simulink model "Motor_Diesel_paC"  (R2017a)
settings: Solver=FixedStepAuto  StartTime=0.0  StopTime=1000  FixedStep=0.01  RelTol=1e-3  EnableMultiTasking=on
undefined symbols (not defined in the file): H_act_d, K1
settings Model: Creator=dmartinez  LastModifiedBy=Administrador
settings OptimizationCC: DefaultParameterBehavior=Inlined  PassReuseOutputArgsAs=Individual arguments
settings DebuggingCC: ParameterTunabilityLossMsg=error  SFUnexpectedBacktrackingDiag=warning  SFNoUnconditionalDefaultTransitionDiag=warning  SFExecutionAtInitializationDiag=none
settings SFSimCC: MATLABDynamicMemAlloc=off
settings RTWCC: SystemTargetFile=ert.tlc  TemplateMakefile=ert_default_tmf  Description=Embedded Coder  GenerateReport=on  Toolchain=GNU GCC Raspberry Pi  IncludeHyperlinkInReport=on  LaunchReport=on  GenerateTraceInfo=on  GenerateTraceReport=on  GenerateTraceReportSl=on  GenerateTraceReportSf=on  GenerateTraceReportEml=on
settings CodeAppCC: ForceParamTrailComments=on  IgnoreCustomStorageClasses=off  OperatorAnnotations=on  SimulinkDataObjDesc=on  SFDataObjDesc=on  MATLABFcnDesc=on  InsertBlockDesc=on  MATLABSourceComments=on
settings ERTTargetCC: GenerateSampleERTMain=on  InlinedParameterPlacement=NonHierarchical  ERTCustomFileTemplate=example_file_process.tlc
settings ConfigComp: CovMetricSettings=dw  CovHtmlReporting=on  CovSaveCumulativeToWorkspaceVar=on  CovSaveSingleToWorkspaceVar=on  CovExternalEMLEnable=off

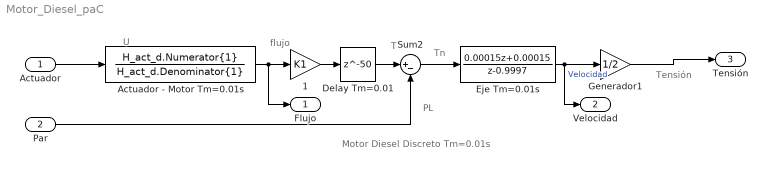
== system Motor_Diesel_paC ==
  note: flujo
  note: T
  note: U
  note: PL
  note: Tn
  note: Motor Diesel Discreto Tm=0.01s
  note: Tensión
  Actuador : Inport  SampleTime=0.01
  Par : Inport  Port=2  SampleTime=0.01
  " 1" : Gain  Gain=K1
  " Generador1" : Gain  Gain=1/2
  Actuador - Motor Tm=0.01s : DiscreteTransferFcn  Numerator=H_act_d.Numerator{1}  Denominator=H_act_d.Denominator{1}  SampleTime=0.01
  Delay Tm=0.01 : Delay  DelayLength=50  SampleTime=0.01
  Eje Tm=0.01s : DiscreteTransferFcn  Numerator=[0.00015 0.00015]  Denominator=[1 -0.9997]  SampleTime=0.01
  Sum2 : Sum  Inputs=|+-
  Flujo : Outport  SampleTime=0.01
  Velocidad : Outport  Port=2  SampleTime=0.01
  Tensión : Outport  Port=3  SampleTime=0.01
  wires:
  Sum2/1 -> Eje Tm=0.01s/1
  Eje Tm=0.01s/1 -> Velocidad/1, " Generador1"/1  "Velocidad"
  Actuador/1 -> Actuador - Motor Tm=0.01s/1
  " Generador1"/1 -> Tensión/1
  Par/1 -> Sum2/2
  Actuador - Motor Tm=0.01s/1 -> " 1"/1, Flujo/1
  " 1"/1 -> Delay Tm=0.01/1
  Delay Tm=0.01/1 -> Sum2/1
